simulink model "quadrotor_system"  (R2018b)
settings: Solver=VariableStepAuto  StartTime=0.0  StopTime=60  RelTol=1e-3
InitFcn:
  | %%%%%%%%%%%%%%%%%%%%%%%%%%%
  | %                         SYSTEM PARAMETERS               %
  | %%%%%%%%%%%%%%%%%%%%%%%%%%%
  | l = 0.232;             % quadrotor arm length
  | b = 3.13e-5;         % propeller lift
  | d = 7.5e-7;           % propeller resistance
  | m = 0.52;             % total quadrotor mass
  | Ix = 6.228e-3;      % Inertia moment X-axis
  | Iy = 6.228e-3;      % Inertia moment Y-axis
  | Iz = 1.121e-2;       % Inertia moment Z-axis
  | Jr = 6e-5;          % Propeller Inertia moment Z-axis
  | Tad = 0.5;        % drag force on the body movement
  | Rad = 0.02;      % drag force on the body rotation
  | g = 9.81;               % gravity
settings Model: Creator=root  LastModifiedBy=root

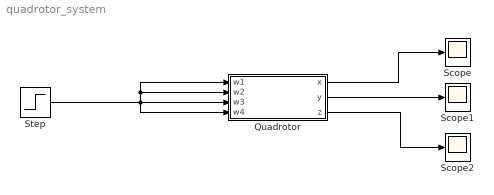
== system quadrotor_system ==
  Quadrotor : Subsystem
  Scope : Scope
  Scope1 : Scope
  Scope2 : Scope
  Step : Step  Time=2  After=7  SampleTime=0
  wires:
  Quadrotor/1(x) -> Scope/1
  Quadrotor/2(y) -> Scope1/1
  Quadrotor/3(z) -> Scope2/1
  Step/1 -> Quadrotor/4(w4), Quadrotor/3(w3), Quadrotor/2(w2), Quadrotor/1(w1)

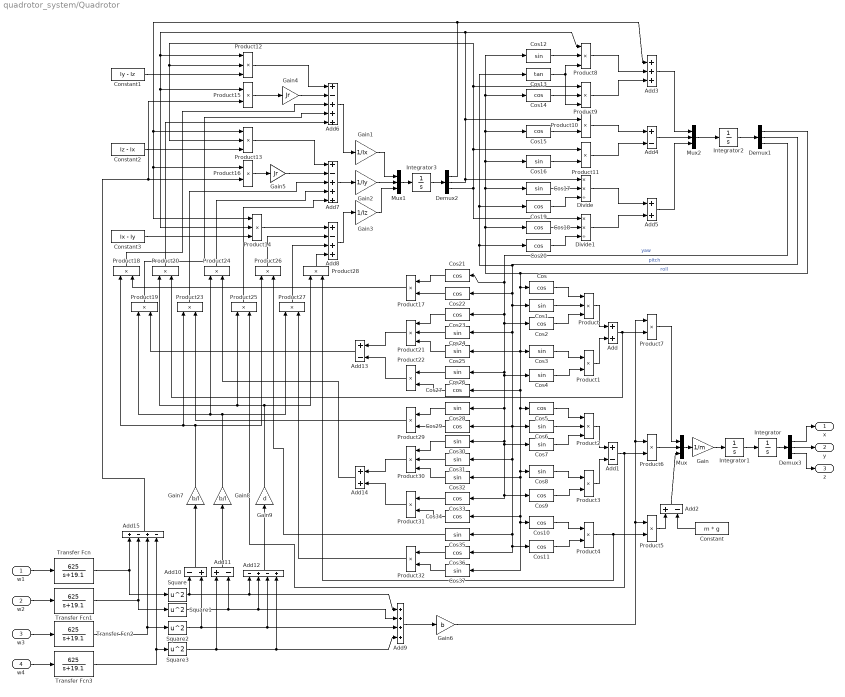
== system quadrotor_system/Quadrotor ==
  w1 : Inport
  w2 : Inport  Port=2
  w3 : Inport  Port=3
  w4 : Inport  Port=4
  Add : Sum
  Add{1..2,4,11,13} (5 alike) : Sum  Inputs=+-
  Add10 : Sum  Inputs=-+
  Add12 : Sum  Inputs=-+-+
  Add14 : Sum
  Add15 : Sum  Inputs=+-+-
  Add3 : Sum  Inputs=+++
  Add5 : Sum
  Add6 : Sum  Inputs=+-+++
  Add7 : Sum  Inputs=+-+++
  Add8 : Sum  Inputs=+-++
  Add9 : Sum  Inputs=++++
  Constant : Constant  Value=m * g
  Constant1 : Constant  Value=Iy - Iz
  Constant2 : Constant  Value=Iz - Ix
  Constant3 : Constant  Value=Ix - Iy
  Cos{,2,5,9..11,14..15,18..23,27,29,33..34,36} (19 alike) : Trigonometry  Operator=cos
  Cos{1,3..4,6..8,12,16..17,24..26,28,30..32,35,37} (18 alike) : Trigonometry
  Cos13 : Trigonometry  Operator=tan
  Demux1 : Demux  Outputs=3
  Demux2 : Demux  Outputs=3
  Demux3 : Demux  Outputs=3
  Divide : Product  Inputs=**/
  Divide1 : Product  Inputs=**/
  Gain : Gain  Gain=1/m
  Gain1 : Gain  Gain=1/Ix
  Gain2 : Gain  Gain=1/Iy
  Gain3 : Gain  Gain=1/Iz
  Gain4 : Gain  Gain=Jr
  Gain5 : Gain  Gain=Jr
  Gain6 : Gain  Gain=b
  Gain7 : Gain  Gain=b/l
  Gain8 : Gain  Gain=b/l
  Gain9 : Gain  Gain=d
  Integrator{,1..3} (4 alike) : Integrator
  Mux : Mux  Inputs=3
  Mux1 : Mux  Inputs=3
  Mux2 : Mux  Inputs=3
  Product{,2,8..9,12..14,21,30} (9 alike) : Product  Inputs=3
  Product{1,3..7,10..11,15..20,22..29,31..32} (24 alike) : Product
  Square{,1..3} (4 alike) : Math  Operator=square  SaturateOnIntegerOverflow=on
  Transfer Fcn{,1..3} (4 alike) : TransferFcn  Numerator=[625]  Denominator=[1 19.1]
  x : Outport
  y : Outport  Port=2
  z : Outport  Port=3
  wires:
  Product7/1 -> Mux/1
  Cos18/1 -> Divide1/2
  Divide/1 -> Add5/1
  Add2/1 -> Mux/3
  Cos15/1 -> Product10/2
  Product10/1 -> Add4/1
  Cos12/1 -> Product8/2
  Product1/1 -> Add/2
  Product11/1 -> Add4/2
  Product8/1 -> Add3/2
  Demux3/1 -> x/1
  Add3/1 -> Mux2/1
  Product5/1 -> Add2/1
  Cos11/1 -> Product4/2
  Add7/1 -> Gain2/1
  Cos17/1 -> Divide/2
  Product/1 -> Add/1
  Cos8/1 -> Product3/1
  Add12/1 -> Gain9/1
  Cos7/1 -> Product2/3
  Add8/1 -> Gain3/1
  Add5/1 -> Mux2/3
  Gain/1 -> Integrator1/1
  Cos19/1 -> Divide/3
  Product4/1 -> Product5/2, Product28/2
  Integrator/1 -> Demux3/1
  Square1/1 -> Add11/2, Add12/2, Add9/2
  Cos14/1 -> Product9/2
  Demux3/3 -> z/1
  Cos/1 -> Product/1
  Divide1/1 -> Add5/2
  Gain4/1 -> Add6/2
  Cos16/1 -> Product11/2
  Product15/1 -> Gain4/1
  Demux2/2 -> Divide/1, Product8/1, Product14/2, Product15/1, Product12/1, Product10/1
  Product14/1 -> Add8/1
  Gain2/1 -> Mux1/2
  Cos1/1 -> Product/2
  Integrator1/1 -> Integrator/1
  Demux3/2 -> y/1
  Gain6/1 -> Product7/1, Product6/1, Product5/1
  Square2/1 -> Add10/2, Add12/3, Add9/3
  Transfer Fcn2/1 -> Add15/3, Square2/1
  Product6/1 -> Mux/2
  Cos9/1 -> Product3/2
  Add6/1 -> Gain1/1
  Add4/1 -> Mux2/2
  Gain5/1 -> Add7/2
  Integrator2/1 -> Demux1/1
  Add10/1 -> Gain7/1
  Cos4/1 -> Product1/2
  Product3/1 -> Add1/2
  Square/1 -> Add10/1, Add12/1, Add9/1
  Add9/1 -> Gain6/1
  Demux2/3 -> Divide1/1, Product11/1, Product9/1, Product13/2, Product12/2
  Transfer Fcn3/1 -> Square3/1, Add15/4
  Gain3/1 -> Mux1/3
  Product16/1 -> Gain5/1
  Gain1/1 -> Mux1/1
  Constant2/1 -> Product13/3
  Cos10/1 -> Product4/1
  Product2/1 -> Add1/1
  Mux2/1 -> Integrator2/1
  Cos20/1 -> Divide1/3
  Demux1/1 -> Cos18/1, Cos17/1, Cos16/1, Cos14/1, Cos12/1, Cos15/1, Cos25/1, Cos27/1, Cos37/1, Cos10/1, Cos34/1, Cos32/1, Cos8/1, Cos5/1, Cos3/1, Cos/1  "roll"
  Cos2/1 -> Product/3
  Add/1 -> Product20/2, Product7/2
  Constant1/1 -> Product12/3
  Integrator3/1 -> Demux2/1
  Demux2/1 -> Add3/1, Product14/1, Product16/1, Product13/1
  Product12/1 -> Add6/1
  Transfer Fcn1/1 -> Square1/1, Add15/2
  Add11/1 -> Gain8/1
  Constant3/1 -> Product14/3
  Mux/1 -> Gain/1
  Cos3/1 -> Product1/1
  Demux1/3 -> Cos23/1, Cos2/1, Cos26/1, Cos28/1, Cos33/1, Cos9/1, Cos7/1, Cos30/1, Cos4/1, Cos21/1  "yaw"
  Product13/1 -> Add7/1
  Product9/1 -> Add3/3
  Demux1/2 -> Cos20/1, Cos19/1, Cos13/1, Cos1/1, Cos24/1, Cos29/1, Cos35/1, Cos36/1, Cos11/1, Cos31/1, Cos6/1, Cos22/1  "pitch"
  Constant/1 -> Add2/2
  Cos13/1 -> Product9/3, Product8/3
  Mux1/1 -> Integrator3/1
  Cos5/1 -> Product2/1
  Cos6/1 -> Product2/2
  Add1/1 -> Product6/2, Product25/2
  Add15/1 -> Product15/2, Product16/2
  Product18/1 -> Add6/3
  Product19/1 -> Add6/4
  Gain8/1 -> Product24/1, Product19/1, Product27/1
  Gain9/1 -> Product28/1, Product25/1, Product20/1
  Product20/1 -> Add6/5
  Cos21/1 -> Product17/1
  Product17/1 -> Product18/2
  Add13/1 -> Product19/2
  Cos22/1 -> Product17/2
  Product21/1 -> Add13/1
  Product22/1 -> Add13/2
  Cos23/1 -> Product21/1
  Cos24/1 -> Product21/2
  Cos25/1 -> Product21/3
  Cos26/1 -> Product22/1
  Cos27/1 -> Product22/2
  Gain7/1 -> Product18/1, Product23/1, Product26/1
  Product23/1 -> Add7/3
  Product24/1 -> Add7/4
  Product25/1 -> Add7/5
  Product26/1 -> Add8/2
  Product27/1 -> Add8/3
  Product28/1 -> Add8/4
  Cos28/1 -> Product29/1
  Cos29/1 -> Product29/2
  Cos30/1 -> Product30/1
  Product31/1 -> Add14/2
  Cos31/1 -> Product30/2
  Cos33/1 -> Product31/1
  Cos34/1 -> Product31/2
  Product30/1 -> Add14/1
  Cos32/1 -> Product30/3
  Add14/1 -> Product24/2
  Cos35/1 -> Product26/2
  Cos36/1 -> Product32/1
  Cos37/1 -> Product32/2
  Product32/1 -> Product27/2
  Product29/1 -> Product23/2
  Transfer Fcn/1 -> Square/1, Add15/1
  Square3/1 -> Add11/1, Add12/4, Add9/4
  w1/1 -> Transfer Fcn/1
  w2/1 -> Transfer Fcn1/1
  w3/1 -> Transfer Fcn2/1
  w4/1 -> Transfer Fcn3/1
